simulink model "program3"  (Simulink 9.0)
settings: Solver=FixedStepAuto  StartTime=0.0  StopTime=76  RelTol=1e-3  EnableMultiTasking=on
values from neighbouring files (symbols this model uses):
  K_PWM = 8.087    [ModelDD.m]
  l = 0.12    [ModelDD.m]
  R = 0.027    [ModelDD.m]
undefined symbols (not defined in the file or in its folder): DiscIntNeverNeededParam
libraries: legoev3lib x4, simulink x2, simulink_need_slupdate x1
settings Model: Creator=ACER  LastModifiedBy=USER  ExtModeTrigDuration=2
settings SolverCC: PositivePriorityOrder=on
settings DataIOCC: SaveFormat=Dataset  ReturnWorkspaceOutputs=on
settings OptimizationCC: PassReuseOutputArgsAs=Individual arguments  LifeSpan=auto  MaxStackSize=64
settings DebuggingCC: UnderspecifiedInitializationDetection=Simplified  MergeDetectMultiDrivingBlocksExec=error  ParameterTunabilityLossMsg=error  SFUnexpectedBacktrackingDiag=error  SFNoUnconditionalDefaultTransitionDiag=error  SFExecutionAtInitializationDiag=warning
settings HardwareCC: ProdLargestAtomicInteger=Long  ProdLargestAtomicFloat=Float  ProdIntDivRoundTo=Zero  ProdEndianess=LittleEndian  ProdHWDeviceType=ARM Compatible->ARM 9
settings ModelReferenceCC: PropagateSignalLabelsOutOfModel=on
settings SFSimCC: SimUseLocalCustomCode=on  MATLABDynamicMemAlloc=off
settings RTWCC: SystemTargetFile=ert.tlc  HardwareBoard=LEGO MINDSTORMS EV3  TLCOptions="-aInlineSetEventsForThisBaseRateFcn=TLC_FALSE -aSuppressMultiTaskScheduler=TLC_FALSE  -aRateBasedStepFcn=0"  TemplateMakefile=ert_default_tmf  Description=Embedded Coder  GenerateReport=on  RTWUseLocalCustomCode=on  Toolchain=Sourcery G++ Lite v2009q3  IncludeHyperlinkInReport=on  LaunchReport=on  GenerateTraceInfo=on  GenerateTraceReport=on  GenerateTraceReportSl=on  GenerateTraceReportSf=on  GenerateTraceReportEml=on
settings MATStruct: className=codertarget.tools.BuildHook  argsTopModelOnly=[]  excludedModels=[]  includeReferencedModels=on  includeTopModel=on  enabled=on  UseCoderTarget=[1]  TargetHardware=LEGO MINDSTORMS EV3  RTOS=Linux  RTOSBaseRateTaskPriority=40  DetectTaskOverruns=[0.0]  Scheduler_interrupt_source=[0.0]  DataVersion=2016.02  IPAddress=codertarget.ev3.internal.getEV3ExtmodeIPaddr  Port=17725  Verbose=[0]  Configuration=TCP/IP  Running=[0.0]  BuildAction=Build, load and run  type=USB  deviceID=0016534b0c89  IPAddressCpy=192.168.43.195
settings CodeAppCC: ForceParamTrailComments=on  IgnoreCustomStorageClasses=off  OperatorAnnotations=on  SimulinkDataObjDesc=on  SFDataObjDesc=on  InsertBlockDesc=on  StateflowObjectComments=off
settings ERTTargetCC: SupportContinuousTime=on  SupportVariableSizeSignals=on
settings ConfigComp: CovMetricSettings=dwe  CovHtmlReporting=off  CovSaveCumulativeToWorkspaceVar=off  CovSaveSingleToWorkspaceVar=off  CovExternalEMLEnable=on

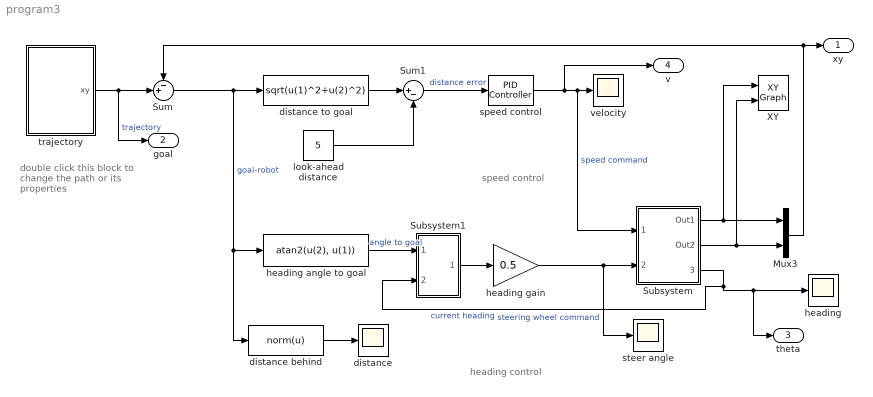
== system program3 ==
  note: double click this block to
      | change the path or its
      | properties
  note: speed control
  note: heading control
  Mux3 : Mux  Inputs=2
  Subsystem : Subsystem
  Subsystem1 : Subsystem
  Sum : Sum  Inputs=-+|
  Sum1 : Sum  Inputs=|+-
  XY : simulink/Sinks/XY Graph  xmin=0  xmax=100  ymin=0  ymax=100  st=-1
  distance : Scope
  distance behind : MATLABFcn  MATLABFcn=norm(u)
  distance to goal : Fcn  Expr=sqrt(u(1)^2+u(2)^2)
  "heading " : Scope
  heading angle to goal : Fcn  Expr=atan2(u(2), u(1))
  heading gain : Gain  Gain=0.5
  look-ahead distance : Constant  Value=5
  speed control : simulink_need_slupdate/PID Controller  P=1  I=0.1  D=0
      settings: SourceProductName=Simulink
  steer angle : Scope
  trajectory : Subsystem  mask(Trajectory generator){path=|, vaxis=[2.5 2.5], tseg=[], dt=0.1, tacc=0, setsimtime=on}
      mask path=|
      | [  10 10;
      |   10 60;
      |   80 80;
      |   50 10 ]
      mask prompts: vaxis "Axis velocities"; tseg "Segment times"; dt "Sample interval"; tacc "Acceleration time"; setsimtime "Set Simulink simulation time"
      mask help: Generate an n-dimensional trajectory using the Toolbox function mstraj.
      mask init:
      | robot_traj = mstraj(path(2:end,:), vaxis, tseg, path(1,:), dt, tacc);
      | total_time = size(robot_traj,1)*dt;
      | if setsimtime
      |     set_param(gcs, 'StopTime', num2str(total_time));
      | end
      mask Help:
      | The trajectory requires a number of parameters
      | 
      | Path: an MxN matrix that defines a path with M points (start, intermediate, goal) and each point is defined by an N-dimensional vector.
      | 
      | Axis velocities: a 1xM vector that specifies the maximum speed of each motion for each dimension.
      | 
      | Segment times: a 1x(N-1) vector of times to execute each motion segment.
      | 
      | Sample time: a scalar sampling time, the trajectory is computed at discrete times with this separation.
      | 
      | Acceleration time: a scalar giving the period of acceleration at each waypoint, as the motion accelerates from one segment to the next.  Can be zero.
      | 
      | This block sets the Simulink simulation time to the length of the trajectory.
      mask Display: plot(path(:,1), path(:,2))
  velocity : Scope
  xy : Outport
  goal : Outport  Port=2
  theta : Outport  Port=3
  v : Outport  Port=4
  wires:
  distance to goal/1 -> Sum1/1
  heading angle to goal/1 -> Subsystem1/1(In1)  "angle to goal"
  distance behind/1 -> distance/1
  look-ahead distance/1 -> Sum1/2
  Sum/1 -> distance behind/1, heading angle to goal/1, distance to goal/1  "goal-robot"
  heading gain/1 -> Subsystem/2(steering wheel angle), steer angle/1  "steering wheel command"
  Subsystem/3(current heading) -> Subsystem1/2(In2), "heading "/1, theta/1  "current heading"
  trajectory/1(xy) -> goal/1, Sum/2  "trajectory"
  Sum1/1 -> speed control/1  "distance error"
  Subsystem/1(Out1) -> Mux3/1, XY/1
  Subsystem/2(Out2) -> XY/2, Mux3/2
  speed control/1 -> Subsystem/1(speed command), velocity/1, v/1  "speed command"
  Mux3/1 -> Sum/1, xy/1
  Subsystem1/1(heading error) -> heading gain/1

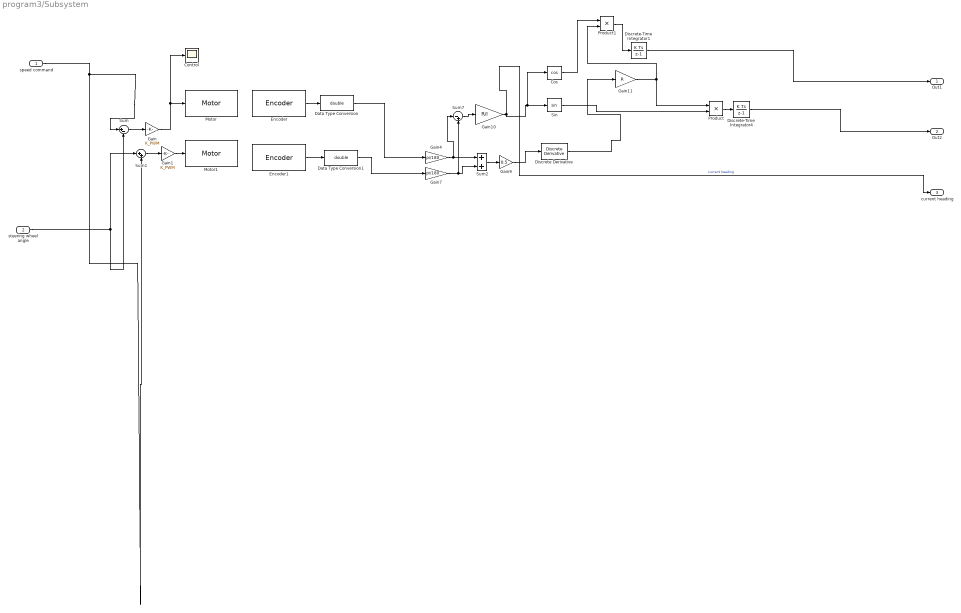
== system program3/Subsystem ==
  speed command : Inport
  steering wheel angle : Inport  Port=2
  Control : Scope
  Cos : Trigonometry  Operator=cos
  Data Type Conversion : DataTypeConversion  OutDataTypeStr=double
  Data Type Conversion1 : DataTypeConversion  OutDataTypeStr=double
  Discrete Derivative : simulink/Discrete/Discrete Derivative  gainval=1.0  ICPrevScaledInput=0.0  OutMin=[]  OutMax=[]  OutDataType=fixdt(1, 16)  OutScaling=2^-10  DoSatur=off
  Discrete-Time Integrator1 : DiscreteIntegrator  InitialConditionSetting=State (most efficient)  SampleTime=0.0033  ICPrevOutput=DiscIntNeverNeededParam  ICPrevScaledInput=DiscIntNeverNeededParam
  Discrete-Time Integrator4 : DiscreteIntegrator  InitialConditionSetting=State (most efficient)  SampleTime=0.0033  ICPrevOutput=DiscIntNeverNeededParam  ICPrevScaledInput=DiscIntNeverNeededParam
  Encoder : legoev3lib/Encoder  portNumber=B  opMode=No reset  sampleTime=Ts
      settings: SourceProductName=Simulink Support Package for LEGO MINDSTORMS EV3 Hardware  SourceProductBaseCode=LEGOEV3
  Encoder1 : legoev3lib/Encoder  portNumber=C  opMode=No reset  sampleTime=Ts
      settings: SourceProductName=Simulink Support Package for LEGO MINDSTORMS EV3 Hardware  SourceProductBaseCode=LEGOEV3
  Gain : Gain  Gain=K_PWM
  Gain1 : Gain  Gain=K_PWM
  Gain10 : Gain  Gain=R/l
  Gain11 : Gain  Gain=R
  Gain4 : Gain  Gain=pi/180
  Gain7 : Gain  Gain=pi/180
  Gain9 : Gain  Gain=0.5
  Motor : legoev3lib/Motor  sportNumber=B  sstopAction=Brake
  Motor1 : legoev3lib/Motor  sportNumber=C  sstopAction=Brake
  Product : Product
  Product1 : Product
  Sin : Trigonometry
  Sum : Sum  Inputs=|+-
  Sum1 : Sum  Inputs=|++
  Sum2 : Sum
  Sum7 : Sum  Inputs=|-+
  Out1 : Outport
  Out2 : Outport  Port=2
  current heading : Outport  Port=3
  wires:
  steering wheel angle/1 -> Sum1/1, Sum/2
  speed command/1 -> Sum1/2, Sum/1
  Discrete-Time Integrator1/1 -> Out1/1
  Gain10/1 -> Cos/1, Sin/1, current heading/1  "current heading"
  Sum7/1 -> Gain10/1
  Gain11/1 -> Product/1, Product1/2
  Product1/1 -> Discrete-Time Integrator1/1
  Gain7/1 -> Sum7/2, Sum2/2
  Discrete Derivative/1 -> Gain11/1
  Gain9/1 -> Discrete Derivative/1
  Product/1 -> Discrete-Time Integrator4/1
  Gain4/1 -> Sum7/1, Sum2/1
  Sin/1 -> Product/2
  Discrete-Time Integrator4/1 -> Out2/1
  Cos/1 -> Product1/1
  Sum2/1 -> Gain9/1
  Sum1/1 -> Gain1/1
  Encoder/1 -> Data Type Conversion/1
  Encoder1/1 -> Data Type Conversion1/1
  Sum/1 -> Gain/1
  Data Type Conversion/1 -> Gain4/1
  Data Type Conversion1/1 -> Gain7/1
  Gain/1 -> Motor/1, Control/1
  Gain1/1 -> Motor1/1

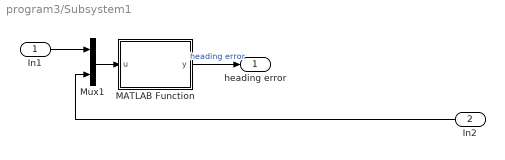
== system program3/Subsystem1 ==
  In1 : Inport
  In2 : Inport  Port=2
  MATLAB Function : MATLAB Function  TreatAsAtomicUnit=on
  Mux1 : Mux  Inputs=2
  heading error : Outport
  wires:
  In2/1 -> Mux1/2
  In1/1 -> Mux1/1
  MATLAB Function/1(y) -> heading error/1  "heading error"
  Mux1/1 -> MATLAB Function/1(u)

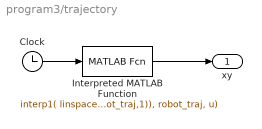
== system program3/trajectory ==
  Clock : Clock
  Interpreted MATLAB Function : MATLABFcn  MATLABFcn=interp1( linspace(0, total_time, size(robot_traj,1)), robot_traj, u)
  xy : Outport
  wires:
  Clock/1 -> Interpreted MATLAB Function/1
  Interpreted MATLAB Function/1 -> xy/1

== matlab function Subsystem1/MATLAB Function ==
  data: u input double; y output double
function y = fcn(u)

y = angdiff(u(2),u(1));
